simulink model "quarter_car_model_passive"  (R2022b)
settings: Solver=VariableStepAuto  StartTime=0.0  StopTime=10.0  RelTol=1e-3
settings Model: Creator=Dharshan K  LastModifiedBy=Dharshan K

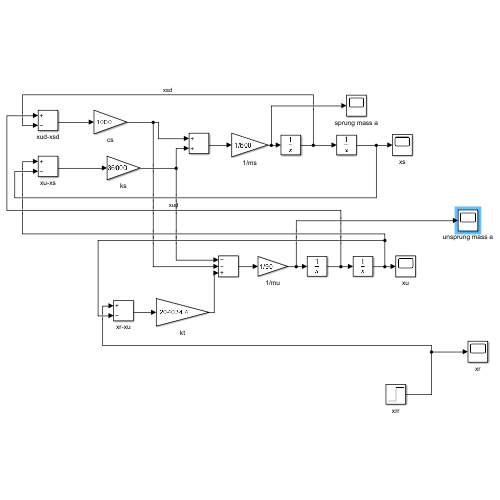
[thumbnail: Simulink's stored preview of the top-level diagram]
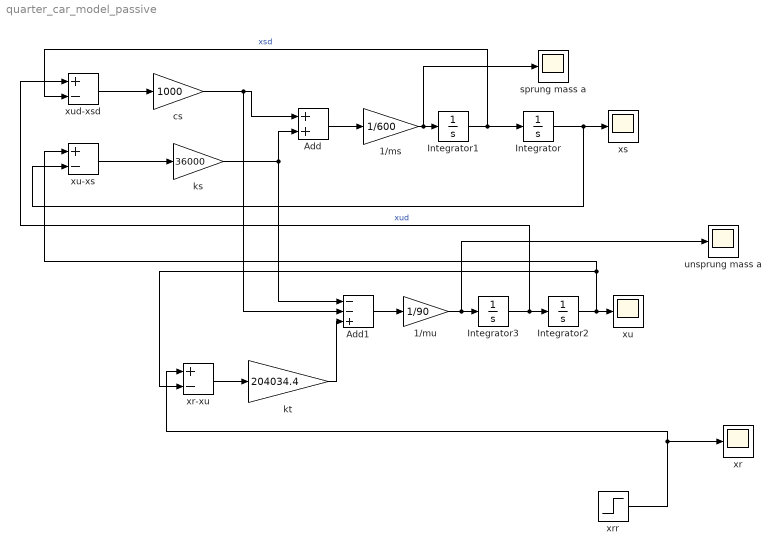
== system quarter_car_model_passive ==
  1/ms : Gain  Gain=1/600
  1/mu : Gain  Gain=1/90
  Add : Sum
  Add1 : Sum  Inputs=--+
  Integrator{,1..3} (4 alike) : Integrator
  cs : Gain  Gain=1000
  ks : Gain  Gain=36000
  kt : Gain  Gain=204034.4
  sprung mass a : Scope
  unsprung mass a : Scope
  xr : Scope
  xr-xu : Sum  Inputs=+-
  xrr : Step  SampleTime=0
  xs : Scope
  xu : Scope
  xu-xs : Sum  Inputs=+-
  xud-xsd : Sum  Inputs=+-
  wires:
  Integrator/1 -> xu-xs/2, xs/1
  Integrator1/1 -> xud-xsd/2, Integrator/1  "xsd"
  1/ms/1 -> sprung mass a/1, Integrator1/1
  Add/1 -> 1/ms/1
  cs/1 -> Add1/2, Add/1
  xud-xsd/1 -> cs/1
  Integrator2/1 -> xr-xu/2, xu-xs/1, xu/1
  Integrator3/1 -> xud-xsd/1, Integrator2/1  "xud"
  xu-xs/1 -> ks/1
  ks/1 -> Add/2, Add1/1
  Add1/1 -> 1/mu/1
  kt/1 -> Add1/3
  xrr/1 -> xr-xu/1, xr/1
  xr-xu/1 -> kt/1
  1/mu/1 -> unsprung mass a/1, Integrator3/1
